simulink model "desc_func1"  (R2025b)
settings: Solver=VariableStepAuto  StartTime=0.0  StopTime=100.0  RelTol=1e-3
settings Model: Creator=Predrag  LastModifiedBy=Predrag

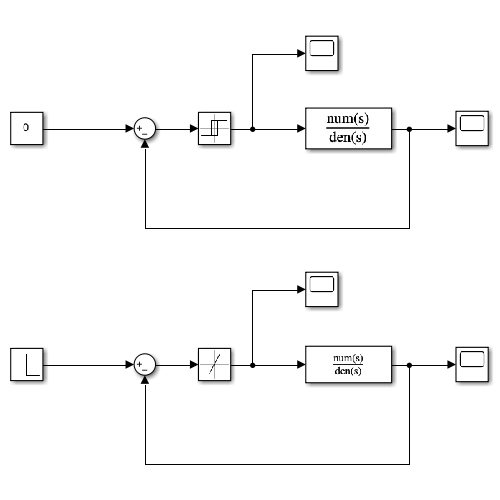
[thumbnail: Simulink's stored preview of the top-level diagram]
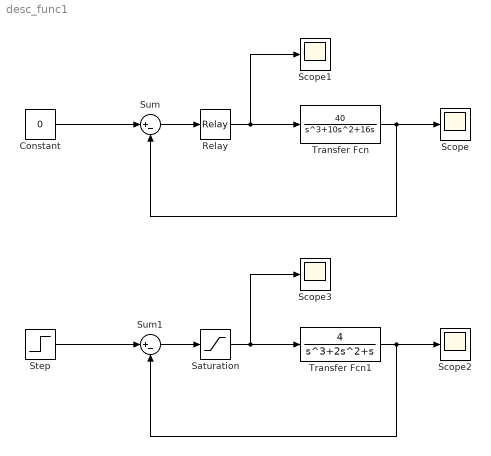
== system desc_func1 ==
  Constant : Constant  Value=0
  Relay : Relay  OnSwitchValue=1  OffSwitchValue=-1  OffOutputValue=-1
  Saturation : Saturate  UpperLimit=1  LowerLimit=-1
  Scope{,1..3} (4 alike) : Scope
      Scope settings: ActiveDisplayYMinimum=-2.0205556682290187  ActiveDisplayYMaximum=2.0205274087391016
      Scope1 settings: ActiveDisplayYMinimum=-1  ActiveDisplayYMaximum=1
      Scope2 settings: ActiveDisplayYMinimum=-2.7839160079592102  ActiveDisplayYMaximum=5.10036345939781  DataLoggingVariableName=ScopeData2
      Scope3 settings: ActiveDisplayYMinimum=-1.25  ActiveDisplayYMaximum=1.25  DataLoggingVariableName=ScopeData3
  Step : Step  Time=10  Before=1  After=0  SampleTime=0
  Sum : Sum  Inputs=|+-
  Sum1 : Sum  Inputs=|+-
  Transfer Fcn : TransferFcn  Numerator=[40]  Denominator=[1 10 16 0]
  Transfer Fcn1 : TransferFcn  Numerator=[4]  Denominator=[1 2 1 0]
  wires:
  Relay/1 -> Scope1/1, Transfer Fcn/1
  Sum/1 -> Relay/1
  Constant/1 -> Sum/1
  Transfer Fcn/1 -> Scope/1, Sum/2
  Transfer Fcn1/1 -> Sum1/2, Scope2/1
  Step/1 -> Sum1/1
  Sum1/1 -> Saturation/1
  Saturation/1 -> Transfer Fcn1/1, Scope3/1
